simulink model "Gateaway_STM32"  (R2025b)
settings: Solver=VariableStepAuto  StartTime=0.0  StopTime=10.0  RelTol=1e-3
libraries: dspsrcs4 x1
settings Model: Creator=strog  LastModifiedBy=strog

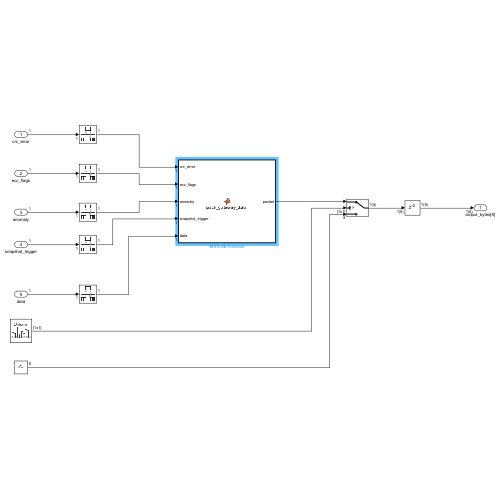
[thumbnail: Simulink's stored preview of the top-level diagram]
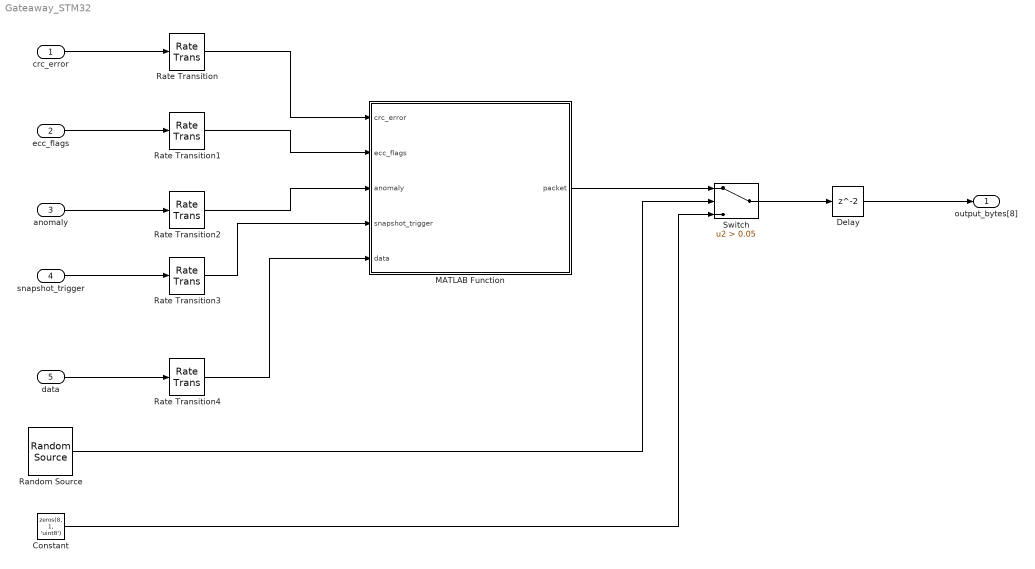
== system Gateaway_STM32 ==
  crc_error : Inport  OutDataTypeStr=boolean
  ecc_flags : Inport  Port=2  OutDataTypeStr=uint8
  anomaly : Inport  Port=3  OutDataTypeStr=boolean
  snapshot_trigger : Inport  Port=4  OutDataTypeStr=boolean
  data : Inport  Port=5  OutDataTypeStr=double
  Constant : Constant  Value=zeros(8, 1, 'uint8')
  Delay : Delay
  MATLAB Function : MATLAB Function  TreatAsAtomicUnit=on
  Random Source : dspsrcs4/Random Source  SrcType=Uniform  MinVal=0  MaxVal=1  MeanVal=0  VarVal=1  RepMode=Specify seed  rawSeed=1  IsInherit=off  SampTime=0.01  SampFrame=1  OutComplex=Real  DataType=double  SimulateUsing=Interpreted execution
  Rate Transition{,1..4} (5 alike) : RateTransition  OutPortSampleTime=0.01
  Switch : Switch  Criteria=u2 > Threshold  Threshold=0.05  SaturateOnIntegerOverflow=off  InputSameDT=off
  output_bytes[8] : Outport
  wires:
  Delay/1 -> output_bytes[8]/1
  MATLAB Function/1(packet) -> Switch/1
  Constant/1 -> Switch/3
  Random Source/1 -> Switch/2
  Switch/1 -> Delay/1
  anomaly/1 -> Rate Transition2/1
  Rate Transition/1 -> MATLAB Function/1(crc_error)
  data/1 -> Rate Transition4/1
  crc_error/1 -> Rate Transition/1
  Rate Transition4/1 -> MATLAB Function/5(data)
  Rate Transition1/1 -> MATLAB Function/2(ecc_flags)
  Rate Transition3/1 -> MATLAB Function/4(snapshot_trigger)
  ecc_flags/1 -> Rate Transition1/1
  Rate Transition2/1 -> MATLAB Function/3(anomaly)
  snapshot_trigger/1 -> Rate Transition3/1

== matlab function Gateaway_STM32/MATLAB Function ==
  data: crc_error input; packet output; ecc_flags input; anomaly input; snapshot_trigger input; data input
function packet = pack_gateway_data(crc_error, ecc_flags, anomaly, snapshot_trigger, data)
%#codegen

% Явно создаем выходной массив байт фиксированного размера
packet = zeros(8, 1, 'uint8');

% Побайтовая упаковка (кодирование) данных
packet(1) = uint8(crc_error);
packet(2) = uint8(ecc_flags);
packet(3) = uint8(anomaly);
packet(4) = uint8(snapshot_trigger);

% Преобразование single (float) в 4 байта uint8 с помощью typecast
data_bytes = typecast(single(data), 'uint8');
packet(5) = data_bytes(1);
packet(6) = data_bytes(2);
packet(7) = data_bytes(3);
packet(8) = data_bytes(4);
end
